simulink model "Project_"  (R2019b)
settings: Solver=ode23tb  StartTime=0.0  StopTime=24*60*60  RelTol=1e-4  AbsTol=5e-3
PreLoadFcn:
  | % Load Data and Parameters used by the model:
  | load power_V2G.mat
  | to=0.1;
undefined symbols (not defined in the file): A, B, C, D1, Dd, Delta, Init, j, V2G
libraries: powerlib x47, simulink x19, powerlib_meascontrol x7, simulink_extras x6, spsDieselMotorModel x1, sps_avr x1, V2Glib x1
(part 1 of 2)
settings Model: SimulationMode=accelerator  ExtModeTrigDuration=100  Creator=MathWorks  LastModifiedBy=mdeat
settings SolverCC: AutoScaleAbsTol=off  MaxConsecutiveMinStep=1e6
settings DataIOCC: LimitDataPoints=on  SaveFormat=Array  ReturnWorkspaceOutputs=off
settings OptimizationCC: BlockReduction=off  BooleanDataType=off  EfficientMapNaN2IntZero=off  LifeSpan=inf
settings DebuggingCC: SaveWithParameterizedLinksMsg=none  UnderspecifiedInitializationDetection=Classic  MergeDetectMultiDrivingBlocksExec=none  SignalResolutionControl=TryResolveAllWithWarning  AllowSymbolicDim=off  SFUnexpectedBacktrackingDiag=warning  SFNoUnconditionalDefaultTransitionDiag=warning  SFExecutionAtInitializationDiag=none  ArithmeticOperatorsInVariantConditions=warning
settings HardwareCC: ProdBitPerPointer=32  ProdBitPerSizeT=32  ProdBitPerPtrDiffT=32  ProdLargestAtomicFloat=None  ProdIntDivRoundTo=Undefined  ProdEndianess=Unspecified  ProdWordSize=32  ProdHWDeviceType=32-bit Generic  TargetBitPerPointer=64  TargetBitPerSizeT=64  TargetBitPerPtrDiffT=64  TargetLongLongMode=on  TargetIntDivRoundTo=Zero  TargetEndianess=LittleEndian  TargetWordSize=64  TargetHWDeviceType=MATLAB Host  ProdEqTarget=off
settings ModelReferenceCC: PropagateSignalLabelsOutOfModel=off
settings SFSimCC: SimUseLocalCustomCode=off  CustomCodeUndefinedFunction=UseInterfaceOnly
settings RTWCC: RTWUseLocalCustomCode=off
settings CodeAppCC: MaxIdLength=128
settings GRTTargetCC: TargetLangStandard=C89/C90 (ANSI)  CombineOutputUpdateFcns=off  GRTInterface=on
settings ConfigComp: CovMetricSettings=dw  CovHtmlReporting=on  CovSaveCumulativeToWorkspaceVar=on  CovSaveSingleToWorkspaceVar=on  CovExternalEMLEnable=off  CovSFcnEnable=off
settings SimscapeCC: SimscapeNormalizeSystem=off

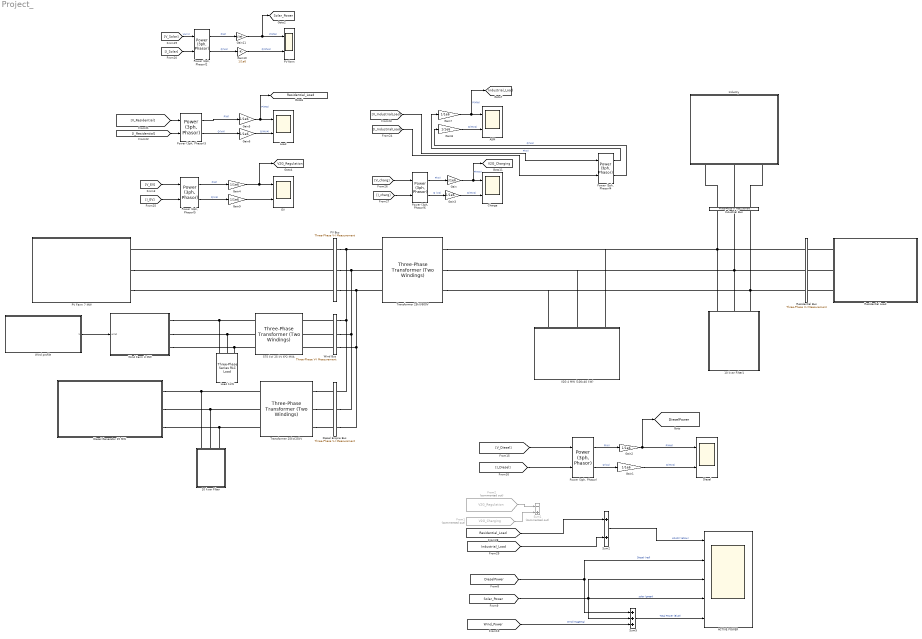
== system Project_ ==
  " Diesel Engine Bus " : powerlib/Measurements/Three-Phase V-I Measurement  VoltageMeasurement=phase-to-ground  SetLabelV=on  LabelV=V_Diesel  Vpu=off  VpuLL=off  CurrentMeasurement=yes  SetLabelI=on  LabelI=I_Diesel  Ipu=off  Pbase=2*1.5e6/0.9  Vbase=25e3  OutputType=Complex  PhasorSimulation=on  PSBequivalent=0
      settings: SourceProductName=Simscape Electrical
  " Industrial Bus" : powerlib/Measurements/Three-Phase V-I Measurement  VoltageMeasurement=phase-to-ground  SetLabelV=on  LabelV=V_IndustrialLoad  Vpu=off  VpuLL=off  CurrentMeasurement=yes  SetLabelI=on  LabelI=I_IndustrialLoad  Ipu=off  Pbase=2*1.5e6/0.9  Vbase=25e3  OutputType=Complex  PhasorSimulation=on  PSBequivalent=0
      settings: SourceProductName=Simscape Electrical
  " Residential Bus" : powerlib/Measurements/Three-Phase V-I Measurement  VoltageMeasurement=phase-to-ground  SetLabelV=on  LabelV=V_Residential  Vpu=off  VpuLL=off  CurrentMeasurement=yes  SetLabelI=on  LabelI=I_Residential  Ipu=off  Pbase=2*1.5e6/0.9  Vbase=25e3  OutputType=Complex  PhasorSimulation=on  PSBequivalent=0
      settings: SourceProductName=Simscape Electrical
  " Wind Bus" : powerlib/Measurements/Three-Phase V-I Measurement  VoltageMeasurement=phase-to-ground  SetLabelV=on  LabelV=V_Wind  Vpu=off  VpuLL=off  CurrentMeasurement=yes  SetLabelI=on  LabelI=I_Wind  Ipu=off  Pbase=6*1.5e6/0.9  Vbase=575  OutputType=Complex  PhasorSimulation=on  PSBequivalent=0
      settings: SourceProductName=Simscape Electrical
  10 kvar Filter : Subsystem
      mask Display: image('$imagefile'); % Use "Edit Image" on toolstrip to change.
  10 kvar Filter1 : Subsystem
      mask Display: image('$imagefile'); % Use "Edit Image" on toolstrip to change.
  575 kV/ 25 kV 6*2 MVA : powerlib/Elements/Three-Phase Transformer (Two Windings)  Winding1Connection=Yg  Winding2Connection=Delta (D1)  CoreType=Three single-phase transformers  SetSaturation=off  Hysteresis=off  DataFile='hysteresis'  SetInitialFlux=off  Measurements=None  UNITS=pu  NominalPower="[6*2e6  60]"  Winding1=[25e3 , 0.025/30 , 0.025]  Winding2=[ 575, 0.025/30 , 0.025]  Rm=500  Lm=inf  L0=0.5  Saturation=[ 0,0 ; 0.0024,1.2 ; 1.0,1.52 ]  InitialFluxes=[ 0.8 , -0.8 , 0.7 ]  BreakLoop=off  DiscreteSolver=Trapezoidal iterative  DataType=off  TransfoNumber=0  mask(Three-Phase Transformer (Two Windings)){}
      settings: SourceProductName=Simscape Electrical
      mask Display: image('$imagefile'); % Use "Edit Image" on toolstrip to change.
  ACTIVE POWER : Scope  NumInputPorts=5
  ASM : Scope  NumInputPorts=2
  Charge : Scope  NumInputPorts=2
  Diesel : Scope  NumInputPorts=2
  Diesel Generator 15 MW : Subsystem
      mask Display: image('$imagefile'); % Use "Edit Image" on toolstrip to change.
  EV : Scope  NumInputPorts=2
  From1 : From  Commented=on  GotoTag=V2G_Charging  TagVisibility=global
  From2 : From  Commented=on  GotoTag=V2G_Regulation  TagVisibility=global
  Gain{,1..11} (12 alike) : Gain  Gain=1/1e6
  Industry : Subsystem
      mask Display: image('$imagefile'); % Use "Edit Image" on toolstrip to change.
  Load : Scope  NumInputPorts=2
  Load 1kW : powerlib/Elements/Three-Phase Series RLC Load  LConnTagsString=A|B|C  Configuration=Y (grounded)  NominalVoltage=(574.706)*1  Vabc=[1e3 1e3 1e3]  Vabcp=[1e3 1e3 1e3]  NominalFrequency=60  UnbalancedPower=off  ActivePower=1e3  InductivePower=0  CapacitivePower=10000  Pabc=[10e3 9e3 11e3]  QLabc=[100 90 110]  QCabc=[100 90 110]  Pabcp=[10e3 9e3 11e3]  QLabcp=[100 90 110]  QCabcp=[100 90 110]  Measurements=None  LoadType=constant PQ
      settings: SourceProductName=Simscape Electrical
  PV Bus : powerlib/Measurements/Three-Phase V-I Measurement  VoltageMeasurement=phase-to-ground  SetLabelV=on  LabelV=V_Solar  Vpu=on  VpuLL=off  CurrentMeasurement=yes  SetLabelI=on  LabelI=I_Solar  Ipu=on  Pbase=2*1.5e6/0.9  Vbase=25e3  OutputType=Complex  PhasorSimulation=on  PSBequivalent=0
      settings: SourceProductName=Simscape Electrical
  PV Farm 7 MW : Subsystem  mask{eff=10, area=8e4}
      mask prompts: eff "Efficiency (%)"; area "Area (m^2)"
      mask help: The product of the effeciency, the area covered by the Pv farm and the irradiance in w/m2 will give you the power generate by the PV farm.
      mask DialogControl DescGroupVar Prompt: PV farm
      mask DialogControl DescTextVar Prompt: The product of the efficiency, the area covered by the PV farm and the irradiance in W/m2 will give you the power generated by the PV farm.
      mask Display: image('house.jpg'); % Use "Edit Image" on toolstrip to change.
  PV farm : Scope  NumInputPorts=2
  Power (3ph, Phasor){,2..6} (6 alike) : powerlib_meascontrol/Measurements/Power (3ph, Phasor)
      settings: SourceProductName=Simscape Electrical  SourceProductBaseCode=PS
  Residential Load : Subsystem  mask{nomPower=10, PF=0.95, timestep=60, datas=V2G.CONSUMPTION}
      mask prompts: nomPower "Nominal Power (MW)"; PF "Power factor"; timestep "Timestep (minutes)"; datas "Consumption datas"
      mask DialogControl DescGroupVar Prompt: Load profile
      mask DialogControl DescTextVar Prompt: The load profile allows you to fix a nominal power and and a power factor. It is also needed to specify the timestep used for the consumption datas. Finally, a vector expresses the consumption profile. It has to be expressed in per unit. It is imperative that the length of the vector fits with the timestep used.
      mask Display: image('$imagefile'); % Use "Edit Image" on toolstrip to change.
  Sum1 : Sum  Commented=on  Inputs=-+
  Sum2 : Sum
  Sum5 : Sum  Inputs=+++
  Transformer 25kV/25kV : powerlib/Elements/Three-Phase Transformer (Two Windings)  Winding1Connection=Delta (D1)  Winding2Connection=Yg  CoreType=Three single-phase transformers  SetSaturation=off  Hysteresis=off  DataFile='hysteresis'  SetInitialFlux=off  Measurements=None  UNITS=pu  NominalPower=[ 20e6 , 60 ]  Winding1=[25e3 , 0.002 , 0.08 ]  Winding2=[ 25e3 , 0.002 , 0.08 ]  Rm=500  Lm=500  L0=0.5  Saturation=[ 0,0 ; 0.0024,1.2 ; 1.0,1.52 ]  InitialFluxes=[ 0.8 , -0.8 , 0.7 ]  BreakLoop=off  DiscreteSolver=Trapezoidal iterative  DataType=off  TransfoNumber=1  mask(Three-Phase Transformer (Two Windings)){}
      settings: SourceProductName=Simscape Electrical
      mask Display: image('$imagefile'); % Use "Edit Image" on toolstrip to change.
  Transformer 25kV/600V : powerlib/Elements/Three-Phase Transformer (Two Windings)  Winding1Connection=Yg  Winding2Connection=Yg  CoreType=Three single-phase transformers  SetSaturation=off  Hysteresis=off  DataFile='hysteresis'  SetInitialFlux=off  Measurements=None  UNITS=pu  NominalPower=[ 20e6 , 60 ]  Winding1=[25e3 ,0.002 , 0.08 ]  Winding2=[ 600 , 0.002 , 0.08 ]  Rm=500  Lm=500  L0=0.5  Saturation=[ 0,0 ; 0.0024,1.2 ; 1.0,1.52 ]  InitialFluxes=[ 0.8 , -0.8 , 0.7 ]  BreakLoop=off  DiscreteSolver=Trapezoidal iterative  DataType=off  TransfoNumber=1  mask(Three-Phase Transformer (Two Windings)){}
      settings: SourceProductName=Simscape Electrical
      mask Display: image('$imagefile'); % Use "Edit Image" on toolstrip to change.
  V2G 4 MW (100x40 kW) : Subsystem  mask{nomPower=20*2, capacity=85, eff=90, enable=on, regGain=[2 4e3], cars1=35, cars2=25, cars3=10, cars4=20, cars5=10}
      mask prompts: nomPower "Rated power (kW)"; capacity "Rated capacity (kWh)"; eff "System efficiency (%)"; enable "V2G on"; regGain "Regulator gain [Kp Ki]"; cars1 "Number of cars  (profile 1)"; cars2 "Number of cars  (profile 2)"; cars3 "Number of cars  (profile 3)"; cars4 "Number of cars  (profile 4)"; cars5 "Number of cars  (profile 5)"
      mask DialogControl DescGroupVar Prompt: V2G
      mask DialogControl DescTextVar Prompt: Models a generic aggregation of electric vehicles. The model has 5 different profiles that can be modified under the mask by changing the plug and the state of charge lookup tables of each profile. The user can set the number of vehicles following each type of profile. The rated capacity, the rated power and the efficiency of the power converter can also be decided by the user. See the example documentation for information about various user profiles.
      mask Display: image('$imagefile'); % Use "Edit Image" on toolstrip to change.
  Wind Farm 3 MW : Subsystem  mask{nomPower=4.5, nomwind=13.5, maxwind=15}
      mask prompts: nomPower "Nominal power (MW)"; nomwind "Nominal wind speed (m/s)"; maxwind "Maximal wind speed (m/s)"
      mask DialogControl DescGroupVar Prompt: Wind farm
      mask DialogControl DescTextVar Prompt: The simplified wind farm model presented here generates power using a linear relationship between the nominal wind speed and nominal power. When the wind speed reaches the maximal value, the wind farm trips from the grid. When the wind speed is between the nominal speed and the maximal value, the power is fixed to 1 p.u.
      mask Display: image('$imagefile'); % Use "Edit Image" on toolstrip to change.
  Wind profile : Subsystem
      mask init:
      | load power_V2G
      mask Display: image('$imagefile'); % Use "Edit Image" on toolstrip to change.
  tag scope: DieselPower=global, Industrial_Load=global, Residential_Load=global, Solar_Power=global, V2G_Charging=global, V2G_Regulation=global
  wires:
  Wind profile/1(" ") -> Wind Farm 3 MW/1(wind)
  [Wind_Power] -> Sum5/3  "Wind (Magenta)"
  [DieselPower] -> ACTIVE POWER/2, Sum5/1  "Diesel (red)"
  [Solar_Power] -> ACTIVE POWER/3, Sum5/2, ACTIVE POWER/4  "solar (green)"
  Sum2/1 -> ACTIVE POWER/1  "LOAD (Yellow)"
  [Industrial_Load] -> Sum2/2
  From1/1 -> Sum1/2
  From2/1 -> Sum1/1
  [I_Diesel] -> "Power (3ph, Phasor)"/2
  Gain2/1 -> [DieselPower], Diesel/1  "P(MW)"
  [V_Diesel] -> "Power (3ph, Phasor)"/1
  "Power (3ph, Phasor)"/1 -> Gain2/1  "P(W)"
  "Power (3ph, Phasor)"/2 -> Gain1/1  "Q(VA)"
  [I_Residential] -> "Power (3ph, Phasor)3"/2
  Gain5/1 -> Load/1, [Residential_Load]  "P(MW)"
  Gain6/1 -> Load/2  "Q(MVA)"
  [V_Residential] -> "Power (3ph, Phasor)3"/1
  "Power (3ph, Phasor)3"/1 -> Gain5/1  "P(W)"
  "Power (3ph, Phasor)3"/2 -> Gain6/1  "Q(VA)"
  "Power (3ph, Phasor)4"/1 -> Gain7/1  "P(W)"
  [V_IndustrialLoad] -> "Power (3ph, Phasor)4"/1
  Gain8/1 -> ASM/2  "Q(MVA)"
  [I_IndustrialLoad] -> "Power (3ph, Phasor)4"/2
  "Power (3ph, Phasor)4"/2 -> Gain8/1  "Q(VA)"
  Gain7/1 -> [Industrial_Load], ASM/1  "P(MW)"
  Gain9/1 -> EV/2
  Gain4/1 -> [V2G_Regulation], EV/1
  "Power (3ph, Phasor)5"/1 -> Gain4/1  "P(W)"
  Gain3/1 -> Charge/2  "Q(MVA)"
  "Power (3ph, Phasor)6"/1 -> Gain/1  "P(W)"
  [I_EV] -> "Power (3ph, Phasor)5"/2
  Gain/1 -> [V2G_Charging], Charge/1  "P(MW)"
  [V_EV] -> "Power (3ph, Phasor)5"/1
  "Power (3ph, Phasor)6"/2 -> Gain3/1  "Q (VA)"
  [I_charg] -> "Power (3ph, Phasor)6"/2
  [V_charg] -> "Power (3ph, Phasor)6"/1
  "Power (3ph, Phasor)5"/2 -> Gain9/1  "Q(VA)"
  Gain1/1 -> Diesel/2  "Q(MVA)"
  Sum5/1 -> ACTIVE POWER/5  "Total Power (Blue)"
  Gain11/1 -> [Solar_Power], PV farm/1  "P(MW)"
  Gain10/1 -> PV farm/2  "Q(MVA)"
  "Power (3ph, Phasor)2"/2 -> Gain10/1  "Q(VA)"
  [I_Solar] -> "Power (3ph, Phasor)2"/2
  [V_Solar] -> "Power (3ph, Phasor)2"/1  "Va (V)"
  "Power (3ph, Phasor)2"/1 -> Gain11/1  "P(W)"
  [Residential_Load] -> Sum2/1
  connections:
  " Diesel Engine Bus "/RConn2 -- " Wind Bus"/RConn2 -- PV Bus/RConn2 -- Transformer 25kV/600V/LConn2
  " Diesel Engine Bus "/RConn3 -- " Wind Bus"/RConn3 -- PV Bus/RConn3 -- Transformer 25kV/600V/LConn3
  Diesel Generator 15 MW/RConn1 -- 10 kvar Filter/LConn1 -- Transformer 25kV/25kV/LConn1
  Diesel Generator 15 MW/RConn3 -- 10 kvar Filter/LConn3 -- Transformer 25kV/25kV/LConn3
  Transformer 25kV/600V/LConn1 -- PV Bus/RConn1 -- " Diesel Engine Bus "/RConn1 -- " Wind Bus"/RConn1
  Transformer 25kV/25kV/RConn1 -- " Diesel Engine Bus "/LConn1
  Transformer 25kV/25kV/RConn3 -- " Diesel Engine Bus "/LConn3
  Transformer 25kV/25kV/RConn2 -- " Diesel Engine Bus "/LConn2
  575 kV/ 25 kV 6*2 MVA/RConn2 -- Load 1kW/LConn2 -- Wind Farm 3 MW/RConn2
  Load 1kW/LConn1 -- 575 kV/ 25 kV 6*2 MVA/RConn1 -- Wind Farm 3 MW/RConn1
  Load 1kW/LConn3 -- 575 kV/ 25 kV 6*2 MVA/RConn3 -- Wind Farm 3 MW/RConn3
  " Wind Bus"/LConn3 -- 575 kV/ 25 kV 6*2 MVA/LConn3
  " Wind Bus"/LConn1 -- 575 kV/ 25 kV 6*2 MVA/LConn1
  " Wind Bus"/LConn2 -- 575 kV/ 25 kV 6*2 MVA/LConn2
  10 kvar Filter1/LConn1 -- Transformer 25kV/600V/RConn1 -- V2G 4 MW (100x40 kW)/LConn3 -- " Residential Bus"/LConn1 -- " Industrial Bus"/LConn1
  10 kvar Filter1/LConn2 -- Transformer 25kV/600V/RConn2 -- V2G 4 MW (100x40 kW)/LConn2 -- " Residential Bus"/LConn2 -- " Industrial Bus"/LConn2
  10 kvar Filter1/LConn3 -- Transformer 25kV/600V/RConn3 -- V2G 4 MW (100x40 kW)/LConn1 -- " Industrial Bus"/LConn3 -- " Residential Bus"/LConn3
  Residential Load/LConn1 -- " Residential Bus"/RConn1
  Residential Load/LConn3 -- " Residential Bus"/RConn3
  Residential Load/LConn2 -- " Residential Bus"/RConn2
  " Industrial Bus"/RConn1 -- Industry/RConn1
  " Industrial Bus"/RConn2 -- Industry/RConn2
  " Industrial Bus"/RConn3 -- Industry/RConn3
  PV Bus/LConn1 -- PV Farm 7 MW/RConn1
  PV Farm 7 MW/RConn2 -- PV Bus/LConn2
  PV Farm 7 MW/RConn3 -- PV Bus/LConn3
  Transformer 25kV/25kV/LConn2 -- 10 kvar Filter/LConn2 -- Diesel Generator 15 MW/RConn2

== system Project_/10 kvar Filter ==
  10 kvar Filter : powerlib/Elements/Three-Phase Series RLC Load  LConnTagsString=A|B|C  Configuration=Y (grounded)  NominalVoltage=600  Vabc=[1e3 1e3 1e3]  Vabcp=[1e3 1e3 1e3]  NominalFrequency=50  UnbalancedPower=off  ActivePower=10e3/100  InductivePower=0  CapacitivePower=10e3  Pabc=[10e3 9e3 11e3]  QLabc=[100 90 110]  QCabc=[100 90 110]  Pabcp=[10e3 9e3 11e3]  QLabcp=[100 90 110]  QCabcp=[100 90 110]  Measurements=None  LoadType=constant Z
      settings: SourceProductName=Simscape Electrical
  A : PMIOPort  Side=Left
  B : PMIOPort  Port=2  Side=Left
  C : PMIOPort  Port=3  Side=Left
  connections:
  10 kvar Filter/LConn2 -- B/RConn1
  10 kvar Filter/LConn3 -- C/RConn1
  10 kvar Filter/LConn1 -- A/RConn1

== system Project_/10 kvar Filter1 ==
  10 kvar Filter1 : powerlib/Elements/Three-Phase Series RLC Load  LConnTagsString=A|B|C  Configuration=Y (grounded)  NominalVoltage=(599.595)*1  Vabc=[1e3 1e3 1e3]  Vabcp=[1e3 1e3 1e3]  NominalFrequency=60  UnbalancedPower=off  ActivePower=10e3/100  InductivePower=0  CapacitivePower=10e3  Pabc=[10e3 9e3 11e3]  QLabc=[100 90 110]  QCabc=[100 90 110]  Pabcp=[10e3 9e3 11e3]  QLabcp=[100 90 110]  QCabcp=[100 90 110]  Measurements=None  LoadType=constant Z
      settings: SourceProductName=Simscape Electrical
  A : PMIOPort  Side=Left
  B : PMIOPort  Port=2  Side=Left
  C : PMIOPort  Port=3  Side=Left
  connections:
  10 kvar Filter1/LConn3 -- C/RConn1
  10 kvar Filter1/LConn2 -- B/RConn1
  10 kvar Filter1/LConn1 -- A/RConn1

== system Project_/Diesel Generator 15 MW ==
  Bus Selector : BusSelector  OutputSignals="dq0 components.Stator voltage  vq (pu),dq0 components.Stator voltage  vd (pu),Mechanical.Rotor speed  wm  (pu)"
  Constant1 : Constant
  Constant2 : Constant
  Diesel Engine Governor : spsDieselMotorModel/Diesel Engine Governor  K=29  Tr=[0.01 0.02 0.2]  Ta=[0.25 0.009 0.0384]  Tlim=[0 1.1]  Td=0.024  Pm0=0.007343
      settings: SourceProductName=Simscape Electrical  SourceProductBaseCode=PS
  Excitation System : sps_avr/Excitation System  tr=20e-3  reg=[ 300, 0.001 ]  exc=[ 1, 0 ]  tgr=[ 0, 0 ]  damp=[ 0.001, 0.1 ]  sat=[ 0, 0 ]  lim=[ -11.5, 11.5, 0 ]  v0=[1 1.0072]
      settings: SourceProductName=Simscape Electrical  SourceProductBaseCode=PS
  Ground : Ground
  Rotor speed (p.u.) : Scope
  Synchronous Machine pu Standard : powerlib/Machines/Synchronous Machine pu Standard  PresetModel=No  MechanicalLoad=Mechanical power Pm  ShowDetailedParameters=on  RotorType=Salient-pole  Units=per unit standard parameters  MeasurementBus=off  NominalParameters="[ 15E6  25e3   60]"  Reactances1=[ 1.81, 0.3, 0.23, 1.76, 0.65, 0.25, 0.15 ]  Reactances2="[ 1.305, 0.296, 0.252, 0.474,  0.243,  0.18 ]"  dAxisTimeConstants=Open-circuit  qAxisTimeConstants=Short-circuit  TimeConstants1="[ 4.4849  0.0681  0.1  ]"  TimeConstants2=[ 8.0, 0.03, 1.0, 0.07 ]  TimeConstants3="[  4.49  0.0681  0.0513  ]"  TimeConstants4=[ 8.0, 0.03, 0.3371, 0.0295 ]  TimeConstants5=[ 1.01, 0.053, 0.1 ]  TimeConstants6=[ 1.3201, 0.023, 1.0, 0.07 ]  TimeConstants7=[0.012 0.003 0.003]  TimeConstants8=[ 1.3201, 0.0231, 0.3371, 0.0295 ]  StatorResistance=0.003  Mechanical=[3.7 0 1 ]  PolePairs=20  InitialConditions=[0 -89.802 0.00913935 0.00913935 0.00913935 -36.542 -156.542 83.458 1.00715]  SetSaturation=off  Saturation=[0.6404,0.7127,0.8441,0.9214,0.9956,1.082,1.19,1.316,1.457;0.7,0.7698,0.8872,0.9466,0.9969,1.046,1.1,1.151,1.201]  LoadFlowParameters=[1,0,0,0,0]  TsPowergui=0  TsBlock=-1  IterativeModel=Trapezoidal non iterative  IterativeDiscreteModel=Trapezoidal non iterative  BusType=swing  Pref=0  Qref=0  Qmin=-inf  Qmax=inf  PLF=0  QLF=0
      settings: SourceProductName=Simscape Electrical
  Conn1 : PMIOPort  Side=Right
  Conn2 : PMIOPort  Port=2  Side=Right
  Conn3 : PMIOPort  Port=3  Side=Right
  tag scope: wm=global
  wires:
  Constant1/1 -> Diesel Engine Governor/1
  Excitation System/1 -> Synchronous Machine pu Standard/2
  Bus Selector/1 -> Excitation System/3  "<Stator voltage  vq (pu)>"
  Bus Selector/3 -> [wm], Rotor speed (p.u.)/1, Diesel Engine Governor/2  "<Rotor speed  wm  (pu)>"
  Bus Selector/2 -> Excitation System/2  "<Stator voltage  vd (pu)>"
  Ground/1 -> Excitation System/4
  Synchronous Machine pu Standard/1 -> Bus Selector/1
  Diesel Engine Governor/1 -> Synchronous Machine pu Standard/1
  Constant2/1 -> Excitation System/1
  connections:
  Synchronous Machine pu Standard/RConn1 -- Conn1/RConn1
  Synchronous Machine pu Standard/RConn3 -- Conn3/RConn1
  Synchronous Machine pu Standard/RConn2 -- Conn2/RConn1

== system Project_/Industry ==
  note: Motor is turned on at 3AM
  Asynchronous Machine (customized) : V2Glib/Asynchronous Machine (custom)  RotorType=Squirrel-cage  PresetModel=No  MechanicalLoad=Torque Tm  ShowDetailedParameters=on  ReferenceFrame=Rotor  Units=pu  MeasurementBus=on  NominalParameters=[1.5e+05 600 60]  Stator=[0.01117 0.04832]  Rotor=[0.006 0.04832]  Cage1=[0.01909 0.0397]  Cage2=[0.01909 0.0397]  Lm=2.424  Mechanical=[0.3096 0.01511 2]  PolePairs=2  InitialConditions=[1 0 0 0 0 0 -120 120]  SimulateSaturation=off  Saturation="[0.212,0.4201,0.8125,1.0979,1.4799,2.2457,3.2586,4.5763,6.4763 ;   0.5,0.7,0.9,1,1.1,1.2 ,1.3,1.4,1.5]"  LoadFlowParameters=0  TsPowergui=0  TsBlock=-1  IterativeModel=Trapezoidal non iterative  IterativeDiscreteModel=Trapezoidal non iterative  Pmec=2e6
      settings: SourceProductName=Simscape Electrical  SourceProductBaseCode=PS
  Breakers : powerlib/Elements/Three-Phase Breaker  InitialState=open  SwitchA=on  SwitchB=on  SwitchC=on  SwitchTimes=[ 3*3600] %Motor is turned on at 3AM  External=off  BreakerResistance=0.001  SnubberResistance=1e6  SnubberCapacitance=inf  Measurements=None
      settings: SourceProductName=Simscape Electrical
  Clock : Subsystem
  Gain : Gain  Gain=1.492e5
  Gain3 : Gain  Gain=1.018/(0.9825^2)
  Gain4 : Gain  Gain=1/1e3
  Math Function : Math  Operator=square  SaturateOnIntegerOverflow=on
  P electric (kW) : Display
      settings: Format=bank
  Product : Product
  Rate Limiter1 : RateLimiter  RisingSlewLimit=1e4  FallingSlewLimit=-1e4  SampleTimeMode=inherited
  Rotor speed (p.u.) : Display
      settings: Format=bank
  Te (p.u.) : Display
      settings: Format=bank
  Three-Phase Series RLC Branch : powerlib/Elements/Three-Phase Series RLC Branch  LConnTagsString=A|B|C  RConnTagsString=A|B|C  BranchType=R  Resistance=1  Inductance=1e-3  Capacitance=1e-6  Measurements=None
      settings: SourceProductName=Simscape Electrical
  powergui : powerlib/powergui  Priority=1  SimulationMode=Phasor  SampleTime=50e-6  frequency=60  Iterations=50  frequencyindice=60  Pbase=10e6  ErrMax=0.0001  UnitsV=kV  UnitsW=MW  buscounter=0  FunctionMessages=off  echomessages=off  EnableUseOfTLC=off  CurrentSourceSwitches=off  DisableSnubberDevices=off  DisableRonSwitches=off  DisableVfSwitches=off  DisplayEquations=off  AutomaticDiscreteSolvers=off  SolverType=Tustin  Interpol=off  ExternalGateDelay=off  methode=off  Ts=100  x0status=blocks  SPID=off  SwTol=0  HookPort=off  NonlinearTolerance=0  nMaxIteration=15  ContinueOnMaxIteration=off  RestoreLinks=warning  ResistiveCurrentMeasurement=off  Frange=[0:2:500]  Ylog=off  Xlog=on  ShowGrid=off  save=off  variable=ZData  structure=0  ZoomFFT=off  StartTime=0.0  cycles=1  DisplayStyle=1  fundamental=60  FreqAxis=off  MaxFrequency=1000  frequencyindicesteady=1  RmsSteady=1  display=off
      settings: SourceProductName=Simscape Electrical
  time (h) : Display
      settings: Format=bank
  Conn1 : PMIOPort  Side=Right
  Conn2 : PMIOPort  Port=2  Side=Right
  Conn3 : PMIOPort  Port=3  Side=Right
  wires:
  Asynchronous Machine (customized)/1 -> Rotor speed (p.u.)/1, Math Function/1, Product/1
  Clock/1(" ") -> time (h)/1
  Math Function/1 -> Gain3/1
  Asynchronous Machine (customized)/2 -> Product/2, Te (p.u.)/1
  Gain4/1 -> P electric (kW)/1
  Gain/1 -> Gain4/1
  Rate Limiter1/1 -> Asynchronous Machine (customized)/1
  Gain3/1 -> Rate Limiter1/1
  Product/1 -> Gain/1
  connections:
  Three-Phase Series RLC Branch/LConn1 -- Breakers/LConn1
  Three-Phase Series RLC Branch/LConn3 -- Breakers/LConn3
  Three-Phase Series RLC Branch/RConn2 -- Asynchronous Machine (customized)/LConn2
  Three-Phase Series RLC Branch/LConn2 -- Breakers/LConn2
  Three-Phase Series RLC Branch/RConn1 -- Asynchronous Machine (customized)/LConn1
  Three-Phase Series RLC Branch/RConn3 -- Asynchronous Machine (customized)/LConn3
  Conn2/RConn1 -- Breakers/RConn2
  Conn1/RConn1 -- Breakers/RConn1
  Conn3/RConn1 -- Breakers/RConn3

== system Project_/PV Farm 7 MW ==
  PV Farm : Subsystem
      mask Display: image(imread('panel.jpg'))
  Sun Irradince : Subsystem
      mask Display: image('$imagefile'); % Use "Edit Image" on toolstrip to change.
  A : PMIOPort  Side=Right
  B : PMIOPort  Port=2  Side=Right
  C : PMIOPort  Port=3  Side=Right
  wires:
  Sun Irradince/1(Out1) -> PV Farm/1(irradiance)
  connections:
  PV Farm/RConn2 -- B/RConn1
  PV Farm/RConn1 -- A/RConn1
  PV Farm/RConn3 -- C/RConn1

== system Project_/Residential Load ==
  CSb : powerlib/Electrical Sources/Controlled Current Source  Initialize=on  Source_Type=AC  Amplitude=9355.5  Phase=(2.751-2*pi/3)*180/pi  Frequency=60  Measurements=Current
      settings: SourceProductName=Simscape Electrical
  Csa : powerlib/Electrical Sources/Controlled Current Source  Initialize=on  Source_Type=AC  Amplitude=9355.5  Phase=2.751*180/pi  Frequency=60  Measurements=Current
      settings: SourceProductName=Simscape Electrical
  Series RLC Branch : powerlib/Elements/Series RLC Branch  LConnTagsString=__new0  RConnTagsString=__new0  BranchType=R  Resistance=1e6  Inductance=1e-3  SetiL0=off  InitialCurrent=0  Capacitance=1e-6  Setx0=off  InitialVoltage=0  Measurements=None
      settings: SourceProductName=Simscape Electrical
  Series RLC Branch1 : powerlib/Elements/Series RLC Branch  LConnTagsString=__new0  RConnTagsString=__new0  BranchType=R  Resistance=1e6  Inductance=1e-3  SetiL0=off  InitialCurrent=0  Capacitance=1e-6  Setx0=off  InitialVoltage=0  Measurements=None
      settings: SourceProductName=Simscape Electrical
  Subsystem : Subsystem
  Voltage Measurement1 : powerlib/Measurements/Voltage Measurement  PhasorSimulation=on  OutputType=Complex  PSBequivalent=0
      settings: SourceProductName=Simscape Electrical
  Voltage Measurement2 : powerlib/Measurements/Voltage Measurement  PhasorSimulation=on  OutputType=Complex  PSBequivalent=0
      settings: SourceProductName=Simscape Electrical
  A : PMIOPort  Tag=PMCPort  Side=Left
  B : PMIOPort  Tag=PMCPort  Port=2  Side=Left
  C : PMIOPort  Tag=PMCPort  Port=3  Side=Left
  wires:
  Voltage Measurement1/1 -> [Vab]
  Voltage Measurement2/1 -> [Vbc]
  [Ia] -> Csa/1
  [Ib] -> CSb/1
  connections:
  Series RLC Branch/LConn1 -- A/RConn1 -- Csa/RConn1 -- Voltage Measurement1/LConn1
  Voltage Measurement2/LConn2 -- C/RConn1 -- Series RLC Branch1/RConn1 -- Csa/LConn1 -- CSb/LConn1
  CSb/RConn1 -- Voltage Measurement2/LConn1 -- Voltage Measurement1/LConn2 -- B/RConn1 -- Series RLC Branch1/LConn1 -- Series RLC Branch/RConn1

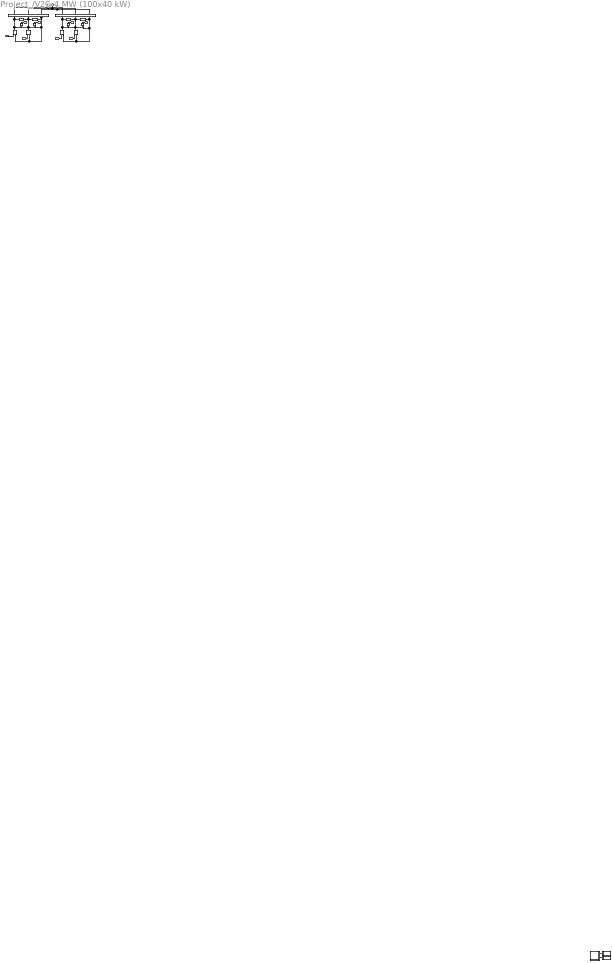
== system Project_/V2G 4 MW (100x40 kW) ==
  " Charge measurement" : powerlib/Measurements/Three-Phase V-I Measurement  VoltageMeasurement=phase-to-ground  SetLabelV=on  LabelV=V_charg  Vpu=off  VpuLL=off  CurrentMeasurement=yes  SetLabelI=on  LabelI=I_charg  Ipu=off  Pbase=2*1.5e6/0.9  Vbase=25e3  OutputType=Complex  PhasorSimulation=on  PSBequivalent=0
      settings: SourceProductName=Simscape Electrical
  " Regulation measurement" : powerlib/Measurements/Three-Phase V-I Measurement  VoltageMeasurement=phase-to-ground  SetLabelV=on  LabelV=V_EV  Vpu=off  VpuLL=off  CurrentMeasurement=yes  SetLabelI=on  LabelI=I_EV  Ipu=off  Pbase=2*1.5e6/0.9  Vbase=25e3  OutputType=Complex  PhasorSimulation=on  PSBequivalent=0
      settings: SourceProductName=Simscape Electrical
  CSb : powerlib/Electrical Sources/Controlled Current Source  Initialize=on  Source_Type=AC  Amplitude=5604.181  Phase=(2.761-2*pi/3)*180/pi  Frequency=60  Measurements=Current
      settings: SourceProductName=Simscape Electrical
  CSb1 : powerlib/Electrical Sources/Controlled Current Source  Initialize=on  Source_Type=AC  Amplitude=5604.181  Phase=(2.761-2*pi/3)*180/pi  Frequency=60  Measurements=Current
      settings: SourceProductName=Simscape Electrical
  Car profiles : Subsystem
  Charge load : Subsystem
  Csa : powerlib/Electrical Sources/Controlled Current Source  Initialize=on  Source_Type=AC  Amplitude=5604.181  Phase=2.761*180/pi  Frequency=60  Measurements=Current
      settings: SourceProductName=Simscape Electrical
  Csa1 : powerlib/Electrical Sources/Controlled Current Source  Initialize=on  Source_Type=AC  Amplitude=5604.181  Phase=2.761*180/pi  Frequency=60  Measurements=Current
      settings: SourceProductName=Simscape Electrical
  Grid regulation : Subsystem
  Series RLC Branch{,1..3} (4 alike) : powerlib/Elements/Series RLC Branch  LConnTagsString=__new0  RConnTagsString=__new0  BranchType=R  Resistance=1e6  Inductance=1e-3  SetiL0=off  InitialCurrent=0  Capacitance=1e-6  Setx0=off  InitialVoltage=0  Measurements=None
      settings: SourceProductName=Simscape Electrical
  Voltage Measurement{1..4} (4 alike) : powerlib/Measurements/Voltage Measurement  PhasorSimulation=on  OutputType=Complex  PSBequivalent=0
      settings: SourceProductName=Simscape Electrical
  "A " : PMIOPort  Tag=PMCPort  Side=Left
  B : PMIOPort  Tag=PMCPort  Port=2  Side=Left
  "C " : PMIOPort  Tag=PMCPort  Port=3  Side=Left
  tag scope: Vab1=global, Vab2=global, Vbc1=global, Vbc2=global
  wires:
  Voltage Measurement1/1 -> [Vab1]
  Voltage Measurement2/1 -> [Vbc1]
  [Ia1] -> Csa/1
  [Ib1] -> CSb/1
  Voltage Measurement3/1 -> [Vab2]
  Voltage Measurement4/1 -> [Vbc2]
  [Ia2] -> Csa1/1
  [Ib2] -> CSb1/1
  Car profiles/1(Cars in regulation) -> Grid regulation/1(Nb_vehicles)
  Car profiles/2(" Cars in charge") -> Charge load/1(Nb_vehicle)
  connections:
  Series RLC Branch/LConn1 -- Csa/RConn1 -- Voltage Measurement1/LConn1 -- " Regulation measurement"/LConn1
  Voltage Measurement2/LConn2 -- Series RLC Branch1/RConn1 -- " Regulation measurement"/LConn3 -- Csa/LConn1 -- CSb/LConn1
  Voltage Measurement1/LConn2 -- " Regulation measurement"/LConn2 -- Series RLC Branch1/LConn1 -- Series RLC Branch/RConn1 -- CSb/RConn1 -- Voltage Measurement2/LConn1
  Voltage Measurement3/LConn1 -- Csa1/RConn1 -- Series RLC Branch2/LConn1 -- " Charge measurement"/RConn1
  Series RLC Branch3/RConn1 -- Csa1/LConn1 -- CSb1/LConn1 -- Voltage Measurement4/LConn2 -- " Charge measurement"/RConn3
  Series RLC Branch3/LConn1 -- Series RLC Branch2/RConn1 -- CSb1/RConn1 -- Voltage Measurement4/LConn1 -- Voltage Measurement3/LConn2 -- " Charge measurement"/RConn2
  " Regulation measurement"/RConn1 -- " Charge measurement"/LConn1 -- "A "/RConn1
  " Regulation measurement"/RConn2 -- " Charge measurement"/LConn2 -- B/RConn1
  " Regulation measurement"/RConn3 -- " Charge measurement"/LConn3 -- "C "/RConn1

== system Project_/Wind Farm 3 MW ==
  note: The wind farm trips around 22h when the
      | wind speed exceeds the maximum wind value
  wind : Inport
  Gain1 : Gain  Gain=1/1e6
  Gain5 : Gain  Gain=1/1e6
  "Power (3ph, Phasor)1" : powerlib_meascontrol/Measurements/Power (3ph, Phasor)
      settings: SourceProductName=Simscape Electrical  SourceProductBaseCode=PS
  Wind Farm : Subsystem
  Wind Farm1 : Scope  NumInputPorts=2
  Wind farm control : Subsystem
  A : PMIOPort  Side=Right
  B : PMIOPort  Port=2  Side=Right
  C : PMIOPort  Port=3  Side=Right
  tag scope: Wind_Power=global
  wires:
  Wind farm control/1(Wind) -> Wind Farm/1("wind ")
  wind/1 -> Wind farm control/1("wind ")
  "Power (3ph, Phasor)1"/1 -> Gain5/1  "P(W)"
  [I_Wind] -> "Power (3ph, Phasor)1"/2
  Gain5/1 -> [Wind_Power], Wind Farm1/1  "P(MW)"
  [V_Wind] -> "Power (3ph, Phasor)1"/1
  "Power (3ph, Phasor)1"/2 -> Gain1/1  "Q(VA)"
  Gain1/1 -> Wind Farm1/2  "Q(MVA)"
  connections:
  Wind Farm/RConn1 -- A/RConn1
  Wind Farm/RConn2 -- B/RConn1
  Wind Farm/RConn3 -- C/RConn1

== system Project_/Wind profile ==
  1-D Lookup Table : Lookup_n-D  NumberOfTableDimensions=1  BreakpointsForDimension1=V2G.WINDTURBINE.time  BeginIndexSearchUsingPreviousIndexResult=on  Table=V2G.WINDTURBINE.wind  ExtrapMethod=Clip  UseLastTableValue=on  InternalRulePriority=Speed  RndMeth=Simplest  InputSameDT=on
  Add : Sum
  Clock1 : Clock
  Constant1 : Constant
  Second-->Hour : Gain  Gain=1/(60*60)
  " " : Outport  VectorParamsAs1DForOutWhenUnconnected=off
  wires:
  Second-->Hour/1 -> Add/1
  Add/1 -> 1-D Lookup Table/1
  Constant1/1 -> Add/2
  Clock1/1 -> Second-->Hour/1
  1-D Lookup Table/1 -> " "/1

== system Project_/Industry/Clock ==
  Clock : Clock
  Gain : Gain  Gain=1/(60*60)
  " " : Outport  VectorParamsAs1DForOutWhenUnconnected=off
  wires:
  Gain/1 -> " "/1
  Clock/1 -> Gain/1

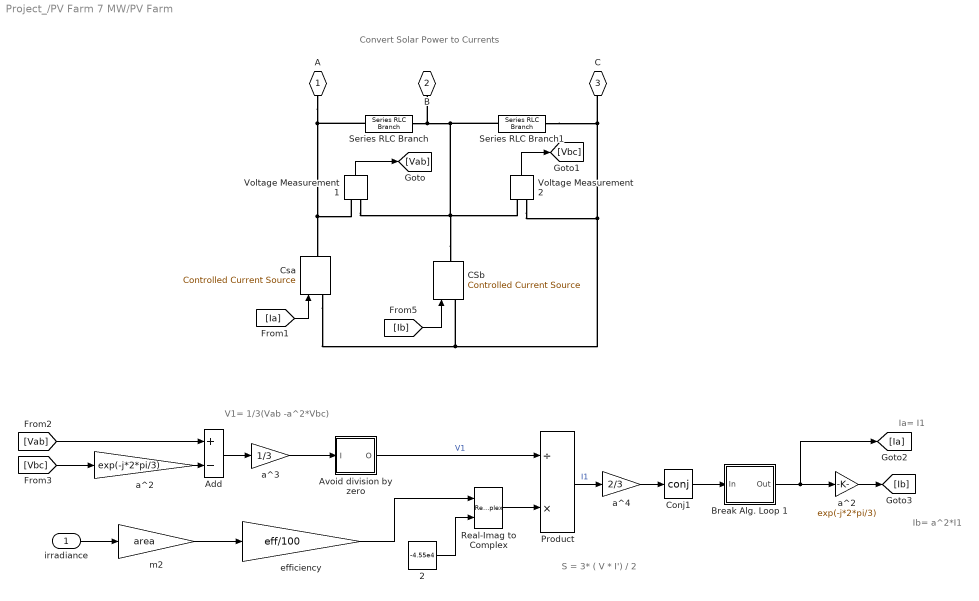
== system Project_/PV Farm 7 MW/PV Farm ==
  note: Ib= a^2*I1
  note: Ia= I1
  note: S = 3* ( V * I') / 2
  note: V1= 1/3(Vab -a^2*Vbc)
  note: Convert Solar Power to Currents
  irradiance : Inport
  2 : Constant  Value=-4.55e4
  Add : Sum  Inputs=+-
  Avoid division by zero : Subsystem
  Break Alg. Loop 1 : Subsystem
  CSb : powerlib/Electrical Sources/Controlled Current Source  Initialize=on  Source_Type=AC  Amplitude=100  Phase=0  Frequency=60  Measurements=None
      settings: SourceProductName=Simscape Electrical
  Conj1 : Math  Operator=conj  SaturateOnIntegerOverflow=on
  Csa : powerlib/Electrical Sources/Controlled Current Source  Initialize=on  Source_Type=AC  Amplitude=100  Phase=0  Frequency=60  Measurements=None
      settings: SourceProductName=Simscape Electrical
  Product : Product  Inputs=/*  SaturateOnIntegerOverflow=on  InputSameDT=on  OutDataTypeStr=Inherit: Same as first input
  Real-Imag to Complex : RealImagToComplex
  Series RLC Branch : powerlib/Elements/Series RLC Branch  LConnTagsString=__new0  RConnTagsString=__new0  BranchType=R  Resistance=1e6  Inductance=1e-3  SetiL0=off  InitialCurrent=0  Capacitance=1e-6  Setx0=off  InitialVoltage=0  Measurements=None
      settings: SourceProductName=Simscape Electrical
  Series RLC Branch1 : powerlib/Elements/Series RLC Branch  LConnTagsString=__new0  RConnTagsString=__new0  BranchType=R  Resistance=1e6  Inductance=1e-3  SetiL0=off  InitialCurrent=0  Capacitance=1e-6  Setx0=off  InitialVoltage=0  Measurements=None
      settings: SourceProductName=Simscape Electrical
  Voltage Measurement1 : powerlib/Measurements/Voltage Measurement  PhasorSimulation=on  OutputType=Complex  PSBequivalent=0
      settings: SourceProductName=Simscape Electrical
  Voltage Measurement2 : powerlib/Measurements/Voltage Measurement  PhasorSimulation=on  OutputType=Complex  PSBequivalent=0
      settings: SourceProductName=Simscape Electrical
  a^2 : Gain  Gain=exp(-j*2*pi/3)  SaturateOnIntegerOverflow=on  OutDataTypeStr=Inherit: Same as input  ParamDataTypeStr=Inherit: Same as input
  "a^2 " : Gain  Gain=exp(-j*2*pi/3)  SaturateOnIntegerOverflow=on  OutDataTypeStr=Inherit: Same as input  ParamDataTypeStr=Inherit: Same as input
  a^3 : Gain  Gain=1/3  SaturateOnIntegerOverflow=on  OutDataTypeStr=Inherit: Same as input  ParamDataTypeStr=Inherit: Same as input
  a^4 : Gain  Gain=2/3  SaturateOnIntegerOverflow=on  OutDataTypeStr=Inherit: Same as input  ParamDataTypeStr=Inherit: Same as input
  efficiency : Gain  Gain=eff/100
  m2 : Gain  Gain=area
  A : PMIOPort  Tag=PMCPort  Side=Right
  B : PMIOPort  Tag=PMCPort  Port=2  Side=Right
  C : PMIOPort  Tag=PMCPort  Port=3  Side=Right
  wires:
  [Ib] -> CSb/1
  Break Alg. Loop 1/1(Out) -> a^2/1, [Ia]
  a^4/1 -> Conj1/1
  "a^2 "/1 -> Add/2
  [Vbc] -> "a^2 "/1
  [Vab] -> Add/1
  Add/1 -> a^3/1
  a^3/1 -> Avoid division by zero/1(I)
  Conj1/1 -> Break Alg. Loop 1/1(In)
  Avoid division by zero/1(O) -> Product/1  "V1"
  a^2/1 -> [Ib]
  [Ia] -> Csa/1
  Product/1 -> a^4/1  "I1"
  Real-Imag to Complex/1 -> Product/2
  Voltage Measurement2/1 -> [Vbc]
  Voltage Measurement1/1 -> [Vab]
  efficiency/1 -> Real-Imag to Complex/1
  2/1 -> Real-Imag to Complex/2
  m2/1 -> efficiency/1
  irradiance/1 -> m2/1
  connections:
  CSb/RConn1 -- Voltage Measurement1/LConn2 -- Voltage Measurement2/LConn1 -- Series RLC Branch/RConn1 -- B/RConn1 -- Series RLC Branch1/LConn1
  Voltage Measurement2/LConn2 -- Csa/LConn1 -- CSb/LConn1 -- C/RConn1 -- Series RLC Branch1/RConn1
  A/RConn1 -- Series RLC Branch/LConn1 -- Voltage Measurement1/LConn1 -- Csa/RConn1

== system Project_/PV Farm 7 MW/Sun Irradince ==
  Irradiance : Subsystem
      mask init:
      | load power_V2G
      mask Display: plot(V2G.IRRADIANCE.time,V2G.IRRADIANCE.SUN)
  Partial Shading : Subsystem  mask(Signal Disturbance){Hour=12, Minute=0, Second=0, Duration=5*60, Factor=0.7}
      mask prompts: Duration "Duration (s):"
      mask help: Within the specified time range defined by Start and Duration parameters, output is set to 'Factor'. Outside the specified time range output is kept at 1.0.
      mask init:
      | T2=(Hour-1)*60*60;    % Hour in seconds
      | T3=(Minute-1)*60;  % Minute in seconds
      | Ton=T2+T3+(Second-1);    % Beginning of fault (s)
      | Toff=Ton+Duration; % End of fault (s)
      mask TypeOptions Hour: 0 |      1 |      2 |      3 |      4 |      5 |      6 |      7 |      8 |      9 |     10 |     11 |     12 |     13 |     14 |     15 |     16 |     17 |     18 |     19 |     20 |     21 |     22 |     23
      mask TypeOptions Minute: 0 |      1 |      2 |      3 |      4 |      5 |      6 |      7 |      8 |      9 |     10 |     11 |     12 |     13 |     14 |     15 |     16 |     17 |     18 |     19 |     20 |     21 |     22 |     23 |     24 |     25 |     26 |     27 |     28 |     29 |     30 |     31 |     32 |     33 |     34 |     35 |     36 |     37 |     38 |     39 |     40 |     41 |     42 |     43 |     44 |     45 |     46 |     47 |     48 |     49 |     50 |     51 |     52 |     53 |     54 |     55 |     56 |     57 |     58 |     59
      mask TypeOptions Second: 0 |      1 |      2 |      3 |      4 |      5 |      6 |      7 |      8 |      9 |     10 |     11 |     12 |     13 |     14 |     15 |     16 |     17 |     18 |     19 |     20 |     21 |     22 |     23 |     24 |     25 |     26 |     27 |     28 |     29 |     30 |     31 |     32 |     33 |     34 |     35 |     36 |     37 |     38 |     39 |     40 |     41 |     42 |     43 |     44 |     45 |     46 |     47 |     48 |     49 |     50 |     51 |     52 |     53 |     54 |     55 |     56 |     57 |     58 |     59
      mask DialogControl Control2 Prompt: Start:
  Product1 : Product
  Rate Limiter2 : RateLimiter  RisingSlewLimit=1e4  FallingSlewLimit=-1e4  SampleTimeMode=inherited
  Out1 : Outport
  wires:
  Partial Shading/1(Out) -> Product1/2
  Product1/1 -> Rate Limiter2/1
  Irradiance/1(" ") -> Product1/1
  Rate Limiter2/1 -> Out1/1

== system Project_/Residential Load/Subsystem ==
  note: Ia= I1
  note: Ib= a^2*I1
  Add : Sum  Inputs=+-
  Avoid division by zero : Subsystem
  Break Alg. Loop 1 : Subsystem
  Conj1 : Math  Operator=conj  SaturateOnIntegerOverflow=on
  Demux : Demux  Outputs=2
  Load : Subsystem
  Product : Product  Inputs=/*  SaturateOnIntegerOverflow=on  InputSameDT=on  OutDataTypeStr=Inherit: Same as first input
  Real-Imag to Complex : RealImagToComplex
  a^2 : Gain  Gain=exp(-j*2*pi/3)  SaturateOnIntegerOverflow=on  OutDataTypeStr=Inherit: Same as input  ParamDataTypeStr=Inherit: Same as input
  "a^2 " : Gain  Gain=exp(-j*2*pi/3)  SaturateOnIntegerOverflow=on  OutDataTypeStr=Inherit: Same as input  ParamDataTypeStr=Inherit: Same as input
  a^3 : Gain  Gain=1/3  SaturateOnIntegerOverflow=on  OutDataTypeStr=Inherit: Same as input  ParamDataTypeStr=Inherit: Same as input
  a^4 : Gain  Gain=2/3  SaturateOnIntegerOverflow=on  OutDataTypeStr=Inherit: Same as input  ParamDataTypeStr=Inherit: Same as input
  wires:
  [Vbc] -> "a^2 "/1
  Product/1 -> a^4/1  "I1"
  "a^2 "/1 -> Add/2
  Demux/1 -> Real-Imag to Complex/1
  a^3/1 -> Avoid division by zero/1(I)
  Load/1(PQ) -> Demux/1
  Real-Imag to Complex/1 -> Product/2
  Break Alg. Loop 1/1(Out) -> [Ia], a^2/1
  Add/1 -> a^3/1
  a^2/1 -> [Ib]
  Avoid division by zero/1(O) -> Product/1  "V1"
  Conj1/1 -> Break Alg. Loop 1/1(In)
  a^4/1 -> Conj1/1
  Demux/2 -> Real-Imag to Complex/2
  [Vab] -> Add/1

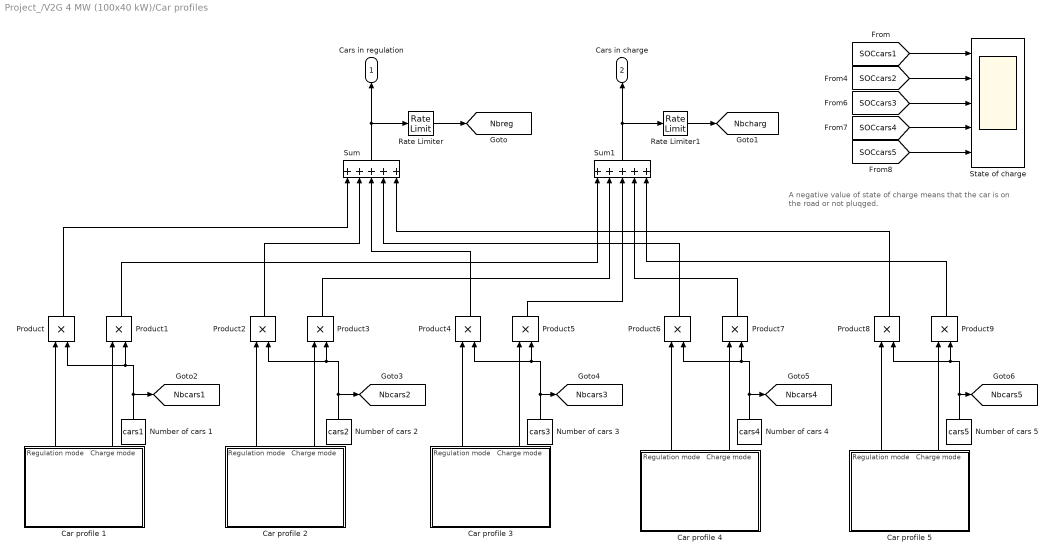
== system Project_/V2G 4 MW (100x40 kW)/Car profiles ==
  note: A negative value of state of charge means that
      | the car is on the road or not pluqged.
  Car profile 1 : Subsystem
  Car profile 2 : Subsystem
  Car profile 3 : Subsystem
  Car profile 4 : Subsystem
  Car profile 5 : Subsystem
  Number of cars 1 : Constant  Value=cars1
  Number of cars 2 : Constant  Value=cars2
  Number of cars 3 : Constant  Value=cars3
  Number of cars 4 : Constant  Value=cars4
  Number of cars 5 : Constant  Value=cars5
  Product{,1..9} (10 alike) : Product
  Rate Limiter : RateLimiter  RisingSlewLimit=10000  FallingSlewLimit=-10000  SampleTimeMode=inherited
  Rate Limiter1 : RateLimiter  RisingSlewLimit=10000  FallingSlewLimit=-10000  SampleTimeMode=inherited
  State of charge : Scope  NumInputPorts=5
  Sum : Sum  Inputs=+++++
  Sum1 : Sum  Inputs=+++++
  Cars in regulation : Outport  VectorParamsAs1DForOutWhenUnconnected=off
  " Cars in charge" : Outport  Port=2  VectorParamsAs1DForOutWhenUnconnected=off
  tag scope: Nbcars1=global, Nbcars2=global, Nbcars3=global, Nbcars4=global, Nbcars5=global, Nbcharg=global, Nbreg=global
  wires:
  Car profile 3/2("Charge mode ") -> Product5/1
  Car profile 2/1("Regulation mode ") -> Product2/1
  Car profile 3/1("Regulation mode ") -> Product4/1
  Car profile 2/2("Charge mode ") -> Product3/1
  Car profile 4/2("Charge mode ") -> Product7/1
  Car profile 4/1("Regulation mode ") -> Product6/1
  Car profile 1/1("Regulation mode ") -> Product/1
  Car profile 1/2("Charge mode ") -> Product1/1
  Number of cars 1/1 -> [Nbcars1], Product1/2, Product/2
  Number of cars 2/1 -> [Nbcars2], Product3/2, Product2/2
  Number of cars 3/1 -> [Nbcars3], Product4/2, Product5/2
  Number of cars 4/1 -> Product6/2, Product7/2, [Nbcars4]
  Number of cars 5/1 -> Product8/2, Product9/2, [Nbcars5]
  Sum/1 -> Cars in regulation/1, Rate Limiter/1
  Sum1/1 -> Rate Limiter1/1, " Cars in charge"/1
  Product/1 -> Sum/1
  Product2/1 -> Sum/2
  Product4/1 -> Sum/3
  Product6/1 -> Sum/4
  Product8/1 -> Sum/5
  Product1/1 -> Sum1/1
  Product3/1 -> Sum1/2
  Product5/1 -> Sum1/3
  Product7/1 -> Sum1/4
  Rate Limiter/1 -> [Nbreg]
  Rate Limiter1/1 -> [Nbcharg]
  Car profile 5/1("Regulation mode ") -> Product8/1
  Car profile 5/2("Charge mode ") -> Product9/1
  Product9/1 -> Sum1/5
  [SOCcars2] -> State of charge/2
  [SOCcars3] -> State of charge/3
  [SOCcars5] -> State of charge/5
  [SOCcars4] -> State of charge/4
  [SOCcars1] -> State of charge/1

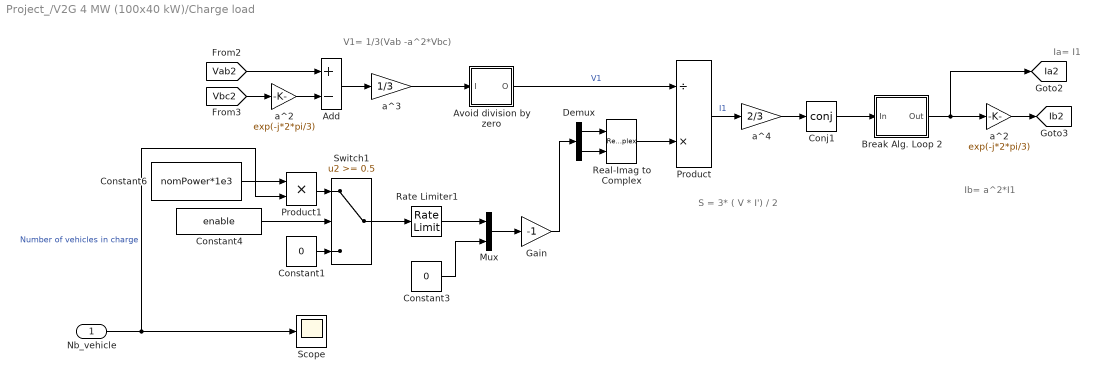
== system Project_/V2G 4 MW (100x40 kW)/Charge load ==
  note: V1= 1/3(Vab -a^2*Vbc)
  note: S = 3* ( V * I') / 2
  note: Ia= I1
  note: Ib= a^2*I1
  Nb_vehicle : Inport
  Add : Sum  Inputs=+-
  Avoid division by zero : Subsystem
  Break Alg. Loop 2 : Subsystem
  Conj1 : Math  Operator=conj  SaturateOnIntegerOverflow=on
  Constant1 : Constant  Value=0
  Constant3 : Constant  Value=0
  Constant4 : Constant  Value=enable
  Constant6 : Constant  Value=nomPower*1e3
  Demux : Demux  Outputs=2
  Gain : Gain  Gain=-1
  Mux : Mux  Inputs=2
  Product : Product  Inputs=/*  SaturateOnIntegerOverflow=on  InputSameDT=on  OutDataTypeStr=Inherit: Same as first input
  Product1 : Product
  Rate Limiter1 : RateLimiter  RisingSlewLimit=1e4  FallingSlewLimit=-1e4  SampleTimeMode=inherited
  Real-Imag to Complex : RealImagToComplex
  Scope : Scope
  Switch1 : Switch  Threshold=0.5  ZeroCross=off
  a^2 : Gain  Gain=exp(-j*2*pi/3)  SaturateOnIntegerOverflow=on  OutDataTypeStr=Inherit: Same as input  ParamDataTypeStr=Inherit: Same as input
  "a^2 " : Gain  Gain=exp(-j*2*pi/3)  SaturateOnIntegerOverflow=on  OutDataTypeStr=Inherit: Same as input  ParamDataTypeStr=Inherit: Same as input
  a^3 : Gain  Gain=1/3  SaturateOnIntegerOverflow=on  OutDataTypeStr=Inherit: Same as input  ParamDataTypeStr=Inherit: Same as input
  a^4 : Gain  Gain=2/3  SaturateOnIntegerOverflow=on  OutDataTypeStr=Inherit: Same as input  ParamDataTypeStr=Inherit: Same as input
  tag scope: Ia2=global, Ib2=global
  wires:
  Real-Imag to Complex/1 -> Product/2
  Product/1 -> a^4/1  "I1"
  a^2/1 -> [Ib2]
  Avoid division by zero/1(O) -> Product/1  "V1"
  Conj1/1 -> Break Alg. Loop 2/1(In)
  a^3/1 -> Avoid division by zero/1(I)
  Add/1 -> a^3/1
  [Vab2] -> Add/1
  [Vbc2] -> "a^2 "/1
  "a^2 "/1 -> Add/2
  a^4/1 -> Conj1/1
  Break Alg. Loop 2/1(Out) -> [Ia2], a^2/1
  Demux/1 -> Real-Imag to Complex/1
  Demux/2 -> Real-Imag to Complex/2
  Gain/1 -> Demux/1
  Rate Limiter1/1 -> Mux/1
  Constant6/1 -> Product1/1
  Nb_vehicle/1 -> Product1/2, Scope/1  "Number of vehicles in charge"
  Constant4/1 -> Switch1/2
  Constant1/1 -> Switch1/3
  Product1/1 -> Switch1/1
  Switch1/1 -> Rate Limiter1/1
  Constant3/1 -> Mux/2
  Mux/1 -> Gain/1

== system Project_/V2G 4 MW (100x40 kW)/Grid regulation ==
  Nb_vehicles : Inport
  Constant : Constant  Value=nomPower*1e3
  Constant2 : Constant  Value=0
  Constant5 : Constant  Value=enable
  Grid regulation ocntrol : Subsystem
  Grid regulation power  generation : Subsystem
  Logical Operator1 : Logic  Operator=NOT  AllPortsSameDT=off  OutDataTypeStr=boolean
  Product : Product
  Rate Limiter2 : RateLimiter  RisingSlewLimit=1e4  FallingSlewLimit=-1e4  SampleTimeMode=inherited
  Scope : Scope
  Switch 2 : Switch  Threshold=0.5  ZeroCross=off
  wires:
  Grid regulation ocntrol/1(PQ) -> Grid regulation power  generation/1("PQ ")
  Constant2/1 -> Switch 2/1
  Switch 2/1 -> Rate Limiter2/1
  Rate Limiter2/1 -> Grid regulation ocntrol/1(Pmax reg)
  Nb_vehicles/1 -> Scope/1, Product/1  "number of vehicles regulator"
  Constant5/1 -> Logical Operator1/1
  Constant/1 -> Product/2
  Product/1 -> Switch 2/3
  Logical Operator1/1 -> Switch 2/2

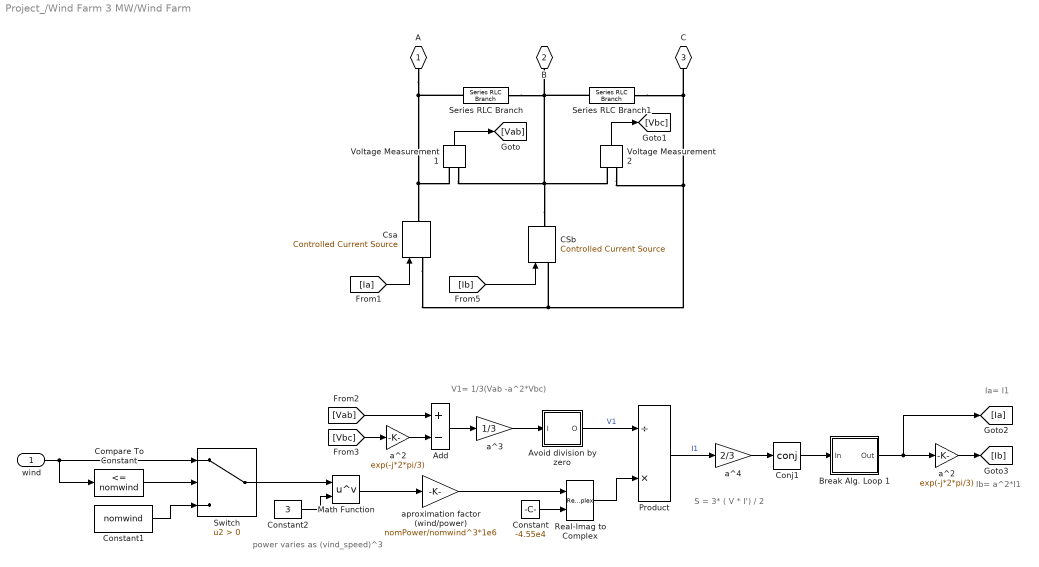
== system Project_/Wind Farm 3 MW/Wind Farm ==
  note: power varies as (vind_speed)^3
  note: V1= 1/3(Vab -a^2*Vbc)
  note: S = 3* ( V * I') / 2
  note: Ia= I1
  note: Ib= a^2*I1
  "wind " : Inport
  Add : Sum  Inputs=+-
  Avoid division by zero : Subsystem
  Break Alg. Loop 1 : Subsystem
  CSb : powerlib/Electrical Sources/Controlled Current Source  Initialize=on  Source_Type=AC  Amplitude=6286.7  Phase=(-0.5-2*pi/3)*180/pi  Frequency=60  Measurements=Current
      settings: SourceProductName=Simscape Electrical
  Compare To Constant : simulink/Logic and Bit Operations/Compare To Constant  relop=<=  const=nomwind  OutDataTypeStr=boolean
  Conj1 : Math  Operator=conj  SaturateOnIntegerOverflow=on
  Constant : Constant  Value=-4.55e4
  Constant1 : Constant  Value=nomwind
  Constant2 : Constant  Value=3
  Csa : powerlib/Electrical Sources/Controlled Current Source  Initialize=on  Source_Type=AC  Amplitude=6286.7  Phase=-0.5*180/pi  Frequency=60  Measurements=Current
      settings: SourceProductName=Simscape Electrical
  Math Function : Math  Operator=pow  SaturateOnIntegerOverflow=on
  Product : Product  Inputs=/*  SaturateOnIntegerOverflow=on  InputSameDT=on  OutDataTypeStr=Inherit: Same as first input
  Real-Imag to Complex : RealImagToComplex
  Series RLC Branch : powerlib/Elements/Series RLC Branch  LConnTagsString=__new0  RConnTagsString=__new0  BranchType=R  Resistance=1e6  Inductance=1e-3  SetiL0=off  InitialCurrent=0  Capacitance=1e-6  Setx0=off  InitialVoltage=0  Measurements=None
      settings: SourceProductName=Simscape Electrical
  Series RLC Branch1 : powerlib/Elements/Series RLC Branch  LConnTagsString=__new0  RConnTagsString=__new0  BranchType=R  Resistance=1e6  Inductance=1e-3  SetiL0=off  InitialCurrent=0  Capacitance=1e-6  Setx0=off  InitialVoltage=0  Measurements=None
      settings: SourceProductName=Simscape Electrical
  Switch : Switch  Criteria=u2 > Threshold
  Voltage Measurement1 : powerlib/Measurements/Voltage Measurement  PhasorSimulation=on  OutputType=Complex  PSBequivalent=0
      settings: SourceProductName=Simscape Electrical
  Voltage Measurement2 : powerlib/Measurements/Voltage Measurement  PhasorSimulation=on  OutputType=Complex  PSBequivalent=0
      settings: SourceProductName=Simscape Electrical
  a^2 : Gain  Gain=exp(-j*2*pi/3)  SaturateOnIntegerOverflow=on  OutDataTypeStr=Inherit: Same as input  ParamDataTypeStr=Inherit: Same as input
  "a^2 " : Gain  Gain=exp(-j*2*pi/3)  SaturateOnIntegerOverflow=on  OutDataTypeStr=Inherit: Same as input  ParamDataTypeStr=Inherit: Same as input
  a^3 : Gain  Gain=1/3  SaturateOnIntegerOverflow=on  OutDataTypeStr=Inherit: Same as input  ParamDataTypeStr=Inherit: Same as input
  a^4 : Gain  Gain=2/3  SaturateOnIntegerOverflow=on  OutDataTypeStr=Inherit: Same as input  ParamDataTypeStr=Inherit: Same as input
  aproximation factor (wind/power) : Gain  Gain=nomPower/nomwind^3*1e6
  A : PMIOPort  Tag=PMCPort  Side=Right
  B : PMIOPort  Tag=PMCPort  Port=2  Side=Right
  C : PMIOPort  Tag=PMCPort  Port=3  Side=Right
  wires:
  "a^2 "/1 -> Add/2
  [Vbc] -> "a^2 "/1
  Avoid division by zero/1(O) -> Product/1  "V1"
  a^3/1 -> Avoid division by zero/1(I)
  Add/1 -> a^3/1
  [Vab] -> Add/1
  aproximation factor (wind/power)/1 -> Real-Imag to Complex/1
  Constant1/1 -> Switch/3
  Compare To Constant/1 -> Switch/2
  "wind "/1 -> Switch/1, Compare To Constant/1
  Constant/1 -> Real-Imag to Complex/2
  Voltage Measurement1/1 -> [Vab]
  Voltage Measurement2/1 -> [Vbc]
  Real-Imag to Complex/1 -> Product/2
  Product/1 -> a^4/1  "I1"
  a^2/1 -> [Ib]
  Conj1/1 -> Break Alg. Loop 1/1(In)
  a^4/1 -> Conj1/1
  Break Alg. Loop 1/1(Out) -> [Ia], a^2/1
  [Ib] -> CSb/1
  [Ia] -> Csa/1
  Math Function/1 -> aproximation factor (wind/power)/1
  Switch/1 -> Math Function/1
  Constant2/1 -> Math Function/2
  connections:
  A/RConn1 -- Csa/RConn1 -- Voltage Measurement1/LConn1 -- Series RLC Branch/LConn1
  Voltage Measurement2/LConn2 -- Series RLC Branch1/RConn1 -- C/RConn1 -- CSb/LConn1 -- Csa/LConn1
  CSb/RConn1 -- Series RLC Branch/RConn1 -- B/RConn1 -- Series RLC Branch1/LConn1 -- Voltage Measurement2/LConn1 -- Voltage Measurement1/LConn2
